simulink library "pureIntegratorWinch_cl"  (R2018b)
settings: Solver=VariableStepAuto  StartTime=0.0  StopTime=10.0  RelTol=1e-3
values from neighbouring files (symbols this model uses):
  initTetherLength = [0 0 0]    [pureIntegrator_ts.m]
  winchMaxSpeed = [5 5 5]    [pureIntegrator_ts.m]
settings Model: Creator=Ayaz  LastModifiedBy=Ayaz

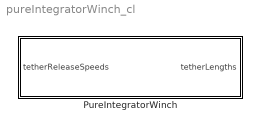
== system pureIntegratorWinch_cl ==
  PureIntegratorWinch : Subsystem  TreatAsAtomicUnit=on  mask{u_max=winchMaxSpeed, iniTetL=initTetherLength}
      mask prompts: u_max "Max winch speed"; iniTetL "Tether initial lengths"

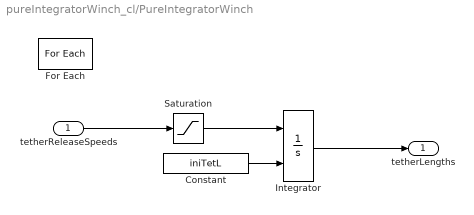
== system pureIntegratorWinch_cl/PureIntegratorWinch ==
  tetherReleaseSpeeds : Inport  Partition=on  PartitionDimension=2  PartitionWidth=1  PartitionOffset=0
  Constant : Constant  Value=iniTetL
  For Each : ForEach  DisableCoverage=on  IterateSubsysMaskParameter=on,on  SubsysMaskParameterIterationDimension=2,2  IndexMode=One-based
  Integrator : Integrator  InitialConditionSource=external
  Saturation : Saturate  UpperLimit=u_max  LowerLimit=-u_max
  tetherLengths : Outport  ConcatenationDimension=2
  wires:
  tetherReleaseSpeeds/1 -> Saturation/1
  Saturation/1 -> Integrator/1
  Integrator/1 -> tetherLengths/1
  Constant/1 -> Integrator/2
